simulink subsystem "sceneHist1"  (R2023a)
settings: Solver=VariableStepAuto  StartTime=0.0  StopTime=10.0  RelTol=1e-3
values from neighbouring files (symbols this model uses):
  Ts = 1/(30*rows*cols)    [LDFItest.m]    (also in LDXItest.m; LXFItest.m; LXFXtest.m; LXXItest.m)
libraries: hdlsllib x1
settings Model: Creator=dileepan  LastModifiedBy=dileepan

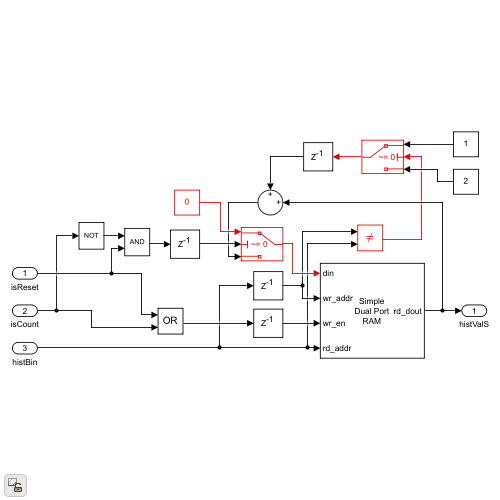
[thumbnail: Simulink's stored preview of the top-level diagram]
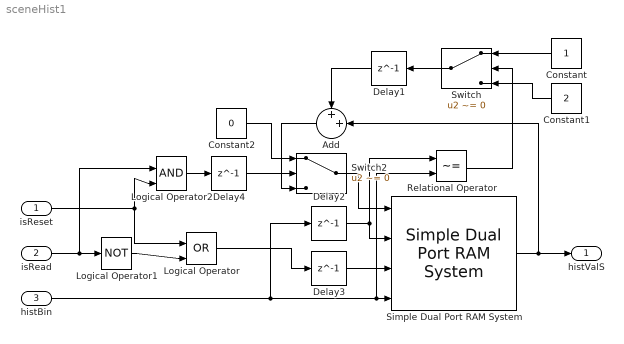
== system sceneHist1 ==
  isReset : Inport
  isRead : Inport  Port=2
  histBin : Inport  Port=3
  Add : Sum  Inputs=++|  AccumDataTypeStr=fixdt(0,ceil(log2(rows*cols)),0)  OutDataTypeStr=Inherit: Same as accumulator
  Constant : Constant  OutDataTypeStr=fixdt(0,2,0)  SampleTime=Ts
  Constant1 : Constant  Value=2  OutDataTypeStr=fixdt(0,2,0)  SampleTime=Ts
  Constant2 : Constant  Value=0  OutDataTypeStr=fixdt(0,ceil(log2(rows*cols)),0)  SampleTime=Ts
  Delay{1..4} (4 alike) : Delay  DelayLength=1
  Logical Operator : Logic  Operator=OR  IconShape=distinctive  AllPortsSameDT=off  OutDataTypeStr=boolean
  Logical Operator1 : Logic  Operator=NOT  IconShape=distinctive  AllPortsSameDT=off  OutDataTypeStr=boolean
  Logical Operator2 : Logic  IconShape=distinctive  AllPortsSameDT=off  OutDataTypeStr=boolean
  Relational Operator : RelationalOperator  Operator=~=  OutDataTypeStr=boolean  RndMeth=Simplest  InputSameDT=off
  Simple Dual Port RAM System : hdlsllib/HDL RAMs/Simple Dual Port RAM System  RAMType=Simple dual port  WriteOutputValue=New data  RAMInitialValue=0  SimulateUsing=Code generation
  Switch : Switch  Criteria=u2 ~= 0  SaturateOnIntegerOverflow=off  InputSameDT=off
  Switch2 : Switch  Criteria=u2 ~= 0  SaturateOnIntegerOverflow=off  InputSameDT=off
  histValS : Outport
  wires:
  isReset/1 -> Logical Operator2/2, Logical Operator/1
  Delay3/1 -> Simple Dual Port RAM System/3
  Delay2/1 -> Relational Operator/1, Simple Dual Port RAM System/2
  histBin/1 -> Delay2/1, Simple Dual Port RAM System/4, Relational Operator/2
  Constant1/1 -> Switch/3
  Logical Operator/1 -> Delay3/1
  Switch2/1 -> Simple Dual Port RAM System/1
  Constant/1 -> Switch/1
  Delay1/1 -> Add/1
  Add/1 -> Switch2/3
  Delay4/1 -> Switch2/2
  Switch/1 -> Delay1/1
  Relational Operator/1 -> Switch/2
  Logical Operator2/1 -> Delay4/1
  Constant2/1 -> Switch2/1
  Logical Operator1/1 -> Logical Operator/2
  isRead/1 -> Logical Operator1/1, Logical Operator2/1
  Simple Dual Port RAM System/1 -> Add/2, histValS/1
